simulink model "joint_impedance_control"  (R2023a)
settings: Solver=FixedStepDiscrete  StartTime=0.0  StopTime=inf  FixedStep=0.001  RelTol=1e-3
PreLoadFcn:
  | frs = FrankaRobotSettings;
libraries: franka_simulink_library x6
settings Model: SimulationMode=external  ExtModeTrigDuration=10000  Creator=vasi_ko  LastModifiedBy=kvasios
settings SolverCC: AlgebraicLoopSolver=TrustRegion
settings DataIOCC: LimitDataPoints=on  SaveFormat=Array  ReturnWorkspaceOutputs=off
settings OptimizationCC: EnhancedBackFolding=on  OptimizeBlockOrder=speed  DifferentSizesBufferReuse=on  OptimizationCustomize=off
settings DebuggingCC: SolverPrmCheckMsg=warning  ParameterTunabilityLossMsg=error  UnconnectedInputMsg=warning  UnconnectedOutputMsg=warning  UnconnectedLineMsg=warning  SFUnexpectedBacktrackingDiag=warning  SFNoUnconditionalDefaultTransitionDiag=warning  SFExecutionAtInitializationDiag=none  ArithmeticOperatorsInVariantConditions=warning
settings ModelReferenceCC: EnableRefExpFcnMdlSchedulingChecks=on  PropagateSignalLabelsOutOfModel=off
settings SFSimCC: SimUseLocalCustomCode=off  MATLABDynamicMemAlloc=off  CustomCodeUndefinedFunction=UseInterfaceOnly  SimTargetLang=C++
settings RTWCC: RTWUseLocalCustomCode=off  BuildConfiguration=Faster Runs  TargetLang=C++  DLArmComputeVersion=19.05
settings CodeAppCC: OperatorAnnotations=on
settings ConfigComp: CovMetricSettings=dw  CovSaveCumulativeToWorkspaceVar=on  CovSaveSingleToWorkspaceVar=on  CovExternalEMLEnable=off  CovSFcnEnable=off

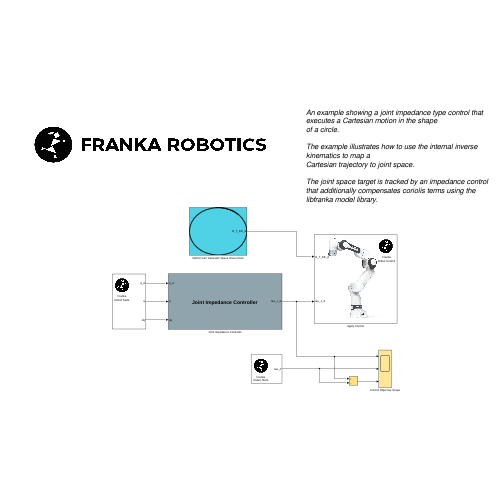
[thumbnail: Simulink's stored preview of the top-level diagram]
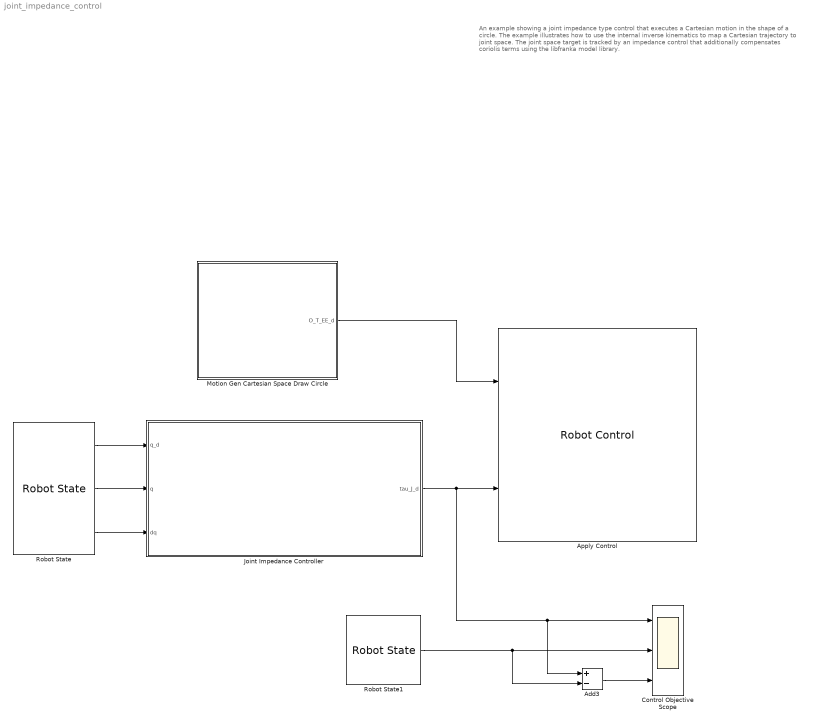
== system joint_impedance_control ==
  note: An example showing a joint impedance type control that executes a Cartesian motion in the shape
      | of a circle.
      |
      | The example illustrates how to use the internal inverse kinematics to map a
      | Cartesian trajectory to joint space.
      |
      | The joint space target is tracked by an impedance control
      | that additionally compensates coriolis terms using the libfranka model library.
  Add3 : Sum  Inputs=+-
  Apply Control : franka_simulink_library/Robot Control  robot_ip=frs.robot_ip  gripper_selection=None  control_mode=Torque Control - Cartesian Pose  controller_choice=Joint Impedance Controller  joint_impedance=[3000, 3000, 3000, 2500, 2500, 2000, 2000]  cartesian_impedance=[3000, 3000, 3000, 300, 300, 300]  rate_limiter=on  cuttoff_frequency=frs.cutoff_frequency  elbow_control=off  collision_thresholds=ones(1,52)*100  load_inertia=frs.load_inertia.getAs1DArray  NE_T_EE=frs.NE_T_EE(:)  EE_T_K=frs.EE_T_K(:)  init_joint_configuration_req=on  init_joint_configuration=frs.home_configuration
      settings: SourceProductName=Franka Robotics Simulink Support Package
  Control Objective Scope : Scope  NumInputPorts=3
  Joint Impedance Controller : Subsystem
      mask Display:
      | disp('{\bf\fontsize{18}Joint Impedance Controller}', 'texmode','on');
      | 
      | block_icon('Controller')
      | 
      | port_label('output',1,'tau_J_d');
      | 
      | port_label('input',1,'q_d');
      | port_label('input',2,'q');
      | port_label('input',3,'dq');
  Motion Gen Cartesian Space Draw Circle : Subsystem
      mask Display:
      | pos = get_param(gcb, 'Position');
      | width = pos(3) - pos(1);
      | x = [0:width];
      | y = sin(x/180*pi);
      | % Parameters 'm' and 'b' must be defined in 'Parameters & Dialog' pane.
      | plot((1/2)*cos(x/180*2*pi+pi/4), (1/2)*sin(x/180*2*pi+pi/4));
      | 
      | port_label('output',1,'O_T_EE_d');
  Robot State : franka_simulink_library/Robot State  robot_ip=frs.robot_ip  signals_requested='q_d q dq'
      settings: SourceProductName=Franka Robotics Simulink Support Package
  Robot State1 : franka_simulink_library/Robot State  robot_ip=frs.robot_ip  signals_requested='tau_J'
      settings: SourceProductName=Franka Robotics Simulink Support Package
  wires:
  Motion Gen Cartesian Space Draw Circle/1(O_T_EE_d) -> Apply Control/1
  Joint Impedance Controller/1(tau_J_d) -> Apply Control/2, Add3/1, Control Objective Scope/1
  Robot State/1 -> Joint Impedance Controller/1(q_d)
  Robot State/2 -> Joint Impedance Controller/2(q)
  Robot State/3 -> Joint Impedance Controller/3(dq)
  Robot State1/1 -> Add3/2, Control Objective Scope/2
  Add3/1 -> Control Objective Scope/3

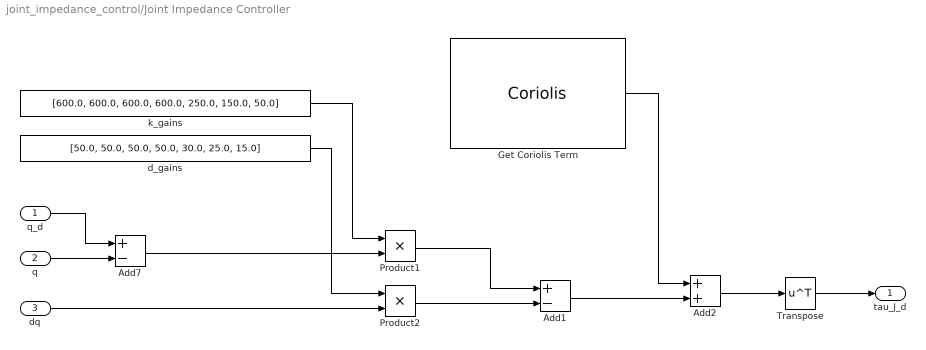
== system joint_impedance_control/Joint Impedance Controller ==
  q_d : Inport
  q : Inport  Port=2
  dq : Inport  Port=3
  Add1 : Sum  Inputs=+-
  Add2 : Sum
  Add7 : Sum  Inputs=+-
  Get Coriolis Term : franka_simulink_library/Coriolis  robot_ip=frs.robot_ip  robot_state_only=on
      settings: SourceProductName=Franka Robotics Simulink Support Package
  Product1 : Product
  Product2 : Product
  Transpose : Math  Operator=transpose
  d_gains : Constant  Value=[50.0, 50.0, 50.0, 50.0, 30.0, 25.0, 15.0]  VectorParams1D=off
  k_gains : Constant  Value=[600.0, 600.0, 600.0, 600.0, 250.0, 150.0, 50.0]  VectorParams1D=off
  tau_J_d : Outport  VectorParamsAs1DForOutWhenUnconnected=off
  wires:
  q_d/1 -> Add7/1
  q/1 -> Add7/2
  k_gains/1 -> Product1/1
  Add7/1 -> Product1/2
  Product1/1 -> Add1/1
  d_gains/1 -> Product2/1
  dq/1 -> Product2/2
  Product2/1 -> Add1/2
  Add2/1 -> Transpose/1
  Add1/1 -> Add2/2
  Transpose/1 -> tau_J_d/1
  Get Coriolis Term/1 -> Add2/1

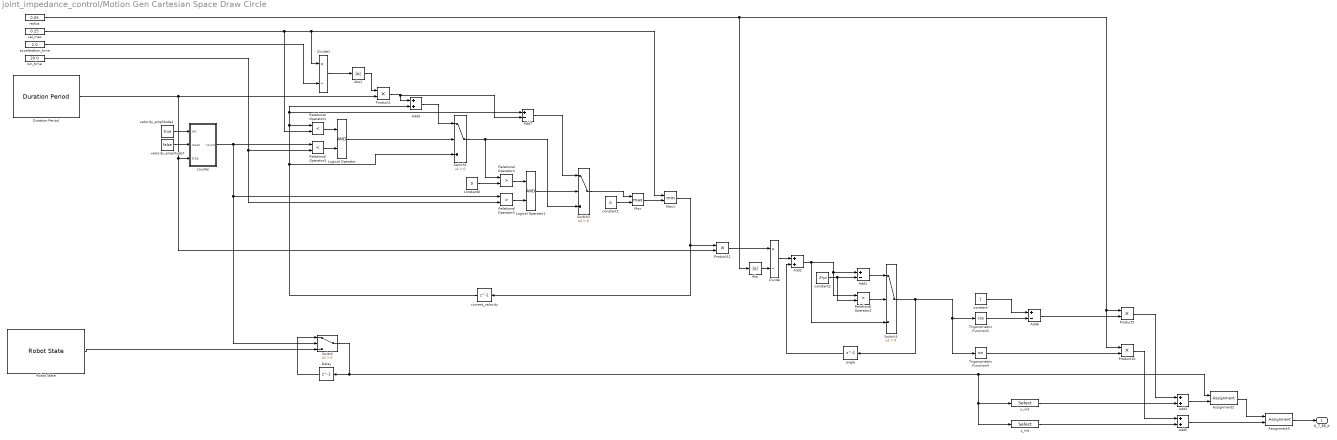
== system joint_impedance_control/Motion Gen Cartesian Space Draw Circle ==
  " Robot State" : franka_simulink_library/Robot State  robot_ip=frs.robot_ip  signals_requested='O_T_EE'
      settings: SourceProductName=Franka Robotics Simulink Support Package
  Abs : Abs  SaturateOnIntegerOverflow=off
  Abs1 : Abs  SaturateOnIntegerOverflow=off
  Add1 : Sum  Inputs=+-
  Add{2..5} (4 alike) : Sum
  Add6 : Sum  Inputs=+-
  Add7 : Sum  Inputs=+-
  Assignment2 : Assignment  DiagnosticForDimensions=Warning  IndexOptions=Index vector (dialog)  Indices=14  OutputSizes=1
  Assignment3 : Assignment  DiagnosticForDimensions=Warning  IndexOptions=Index vector (dialog)  Indices=15  OutputSizes=1
  Delay : Delay  DelayLength=1
  Divide : Product  Inputs=*/
  Divide1 : Product  Inputs=*/
  Duration Period : franka_simulink_library/Duration Period  robot_ip=frs.robot_ip
      settings: SourceProductName=Franka Robotics Simulink Support Package
  Logical Operator : Logic  AllPortsSameDT=off  OutDataTypeStr=boolean
  Logical Operator1 : Logic  AllPortsSameDT=off  OutDataTypeStr=boolean
  Max : MinMax  Function=max  Inputs=2
  Max1 : MinMax  Inputs=2
  Product{1,5,10..11} (4 alike) : Product
  Relational Operator1 : RelationalOperator  Operator=<  OutDataTypeStr=boolean  InputSameDT=off
  Relational Operator2 : RelationalOperator  Operator=>  OutDataTypeStr=boolean  InputSameDT=off
  Relational Operator3 : RelationalOperator  Operator=<  OutDataTypeStr=boolean  InputSameDT=off
  Relational Operator4 : RelationalOperator  Operator=>  OutDataTypeStr=boolean  InputSameDT=off
  Relational Operator5 : RelationalOperator  Operator=>  OutDataTypeStr=boolean  InputSameDT=off
  Switch{,1..3} (4 alike) : Switch  Criteria=u2 > Threshold  SaturateOnIntegerOverflow=off  InputSameDT=off
  Trigonometric Function3 : Trigonometry  Operator=cos  NumberOfIterations=50
  Trigonometric Function4 : Trigonometry  NumberOfIterations=50
  acceleration_time : Constant  Value=2.0  VectorParams1D=off
  angle : Delay  DelayLength=1  InitialCondition=0
  constant : Constant  VectorParams1D=off
  constant0 : Constant  Value=0  VectorParams1D=off
  constant1 : Constant  Value=0  VectorParams1D=off
  constant2 : Constant  Value=2*pi  VectorParams1D=off
  counter : Subsystem
  current_velocity : Delay  DelayLength=1  InitialCondition=0
  radius : Constant  Value=0.05  VectorParams1D=off
  run_time : Constant  Value=20.0  VectorParams1D=off
  vel_max : Constant  Value=0.25  VectorParams1D=off
  velocity_amplitude1 : Constant  Value=true  VectorParams1D=off
  velocity_amplitude7 : Constant  Value=false  VectorParams1D=off
  y_init : Selector  InputPortWidth=16  IndexOptions=Index vector (dialog)  Indices=14  OutputSizes=1
  z_init : Selector  InputPortWidth=16  IndexOptions=Index vector (dialog)  Indices=15  OutputSizes=1
  O_T_EE_d : Outport  VectorParamsAs1DForOutWhenUnconnected=off
  wires:
  Duration Period/1 -> Product11/2, counter/3(step), Product1/2
  velocity_amplitude7/1 -> counter/2(reset)
  velocity_amplitude1/1 -> counter/1(set)
  y_init/1 -> Add4/2
  Add5/1 -> Assignment3/2
  Switch/1 -> z_init/1, y_init/1, Assignment2/1, Delay/1
  Product5/1 -> Add4/1
  z_init/1 -> Add5/2
  Assignment3/1 -> O_T_EE_d/1
  Add4/1 -> Assignment2/2
  Assignment2/1 -> Assignment3/1
  radius/1 -> Product10/1, Product5/1, Abs/1
  Product10/1 -> Add5/1
  Trigonometric Function3/1 -> Add6/2
  constant/1 -> Add6/1
  Add6/1 -> Product5/2
  Trigonometric Function4/1 -> Product10/2
  vel_max/1 -> Max1/1, Divide1/1, Relational Operator1/2
  run_time/1 -> Relational Operator5/2, Relational Operator3/2
  Relational Operator3/1 -> Logical Operator/2
  Relational Operator1/1 -> Logical Operator/1
  Logical Operator/1 -> Switch1/2
  current_velocity/1 -> Switch1/3, Add7/1, Add3/2, Relational Operator1/1
  Logical Operator1/1 -> Switch2/2
  Switch1/1 -> Relational Operator4/1, Switch2/3
  Relational Operator5/1 -> Logical Operator1/2
  Relational Operator4/1 -> Logical Operator1/1
  constant0/1 -> Relational Operator4/2
  Switch2/1 -> Max/1
  constant1/1 -> Max/2
  Max/1 -> Max1/2
  Max1/1 -> current_velocity/1, Product11/1
  Abs/1 -> Divide/2
  Switch3/1 -> angle/1, Trigonometric Function4/1, Trigonometric Function3/1
  Add2/1 -> Relational Operator2/1, Add1/1, Switch3/3
  constant2/1 -> Relational Operator2/2, Add1/2
  Relational Operator2/1 -> Switch3/2
  Add1/1 -> Switch3/1
  Product11/1 -> Divide/1
  angle/1 -> Add2/2
  Divide1/1 -> Abs1/1
  acceleration_time/1 -> Divide1/2
  Abs1/1 -> Product1/1
  Product1/1 -> Add7/2, Add3/1
  Add3/1 -> Switch1/1
  Add7/1 -> Switch2/1
  Divide/1 -> Add2/1
  counter/1(count) -> Switch/2, Relational Operator5/1, Relational Operator3/1
  " Robot State"/1 -> Switch/3
  Delay/1 -> Switch/1

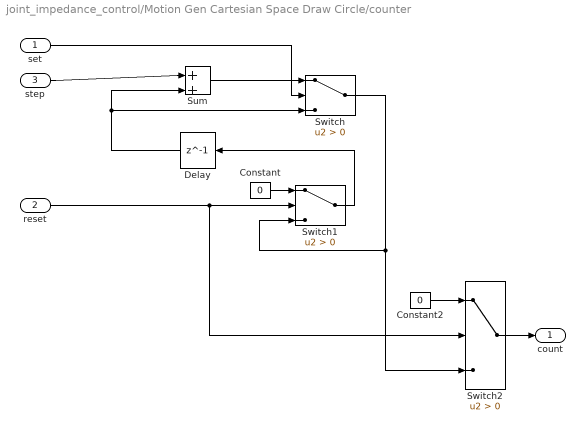
== system joint_impedance_control/Motion Gen Cartesian Space Draw Circle/counter ==
  set : Inport  OutDataTypeStr=boolean
  reset : Inport  Port=2  OutDataTypeStr=boolean
  step : Inport  Port=3  OutDataTypeStr=double
  Constant : Constant  Value=0  OutDataTypeStr=double
  Constant2 : Constant  Value=0  OutDataTypeStr=double
  Delay : Delay  DelayLength=1  InitialCondition=0
  Sum : Sum  Inputs=|++
  Switch : Switch  Criteria=u2 > Threshold  SaturateOnIntegerOverflow=off  InputSameDT=off
  Switch1 : Switch  Criteria=u2 > Threshold  OutDataTypeStr=double  SaturateOnIntegerOverflow=off  InputSameDT=off
  Switch2 : Switch  Criteria=u2 > Threshold  OutDataTypeStr=double  SaturateOnIntegerOverflow=off  InputSameDT=off
  count : Outport  OutDataTypeStr=double  VectorParamsAs1DForOutWhenUnconnected=off
  wires:
  Switch1/1 -> Delay/1
  Constant/1 -> Switch1/1
  reset/1 -> Switch2/2, Switch1/2
  Delay/1 -> Switch/3, Sum/2
  step/1 -> Sum/1
  Switch/1 -> Switch2/3, Switch1/3
  set/1 -> Switch/2
  Sum/1 -> Switch/1
  Constant2/1 -> Switch2/1
  Switch2/1 -> count/1
